simulink model "car"  (R2020a)
settings: Solver=FixedStepDiscrete  StartTime=0.0  StopTime=10.0  FixedStep=0.01  RelTol=1e-3
undefined symbols (not defined in the file or in its folder): f, Gain
libraries: instrumentlib x2
settings Model: Creator=K7050  LastModifiedBy=K7050

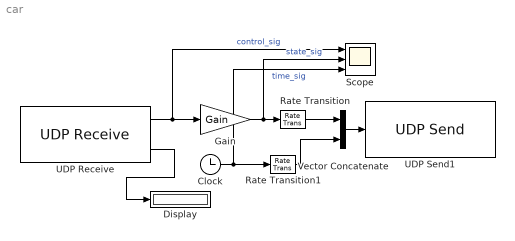
== system car ==
  Clock : Clock
  Display : Display
  Gain : Gain  Gain=Gain
  Rate Transition : RateTransition  OutPortSampleTime=0.01
  Rate Transition1 : RateTransition  OutPortSampleTime=0.01
  Scope : Scope  NumInputPorts=3
  UDP Receive : instrumentlib/UDP Receive  Host=127.0.0.1  Port=12349  LocalPort=12345  EnablePortSharing=off  GetLatestData=off  DataSize=1  DataType=double  ASCIIFormatting=%f,  Terminator=LF  ByteOrder=LittleEndian  EnableBlockingMode=off  Timeout=10  SampleTime=0.01  LocalAddress=127.0.0.1
  UDP Send1 : instrumentlib/UDP Send  Host=127.0.0.1  Port=12346  LocalPort=12351  EnablePortSharing=off  ByteOrder=LittleEndian  OutputDatagramPacketSize=16  EnableBlockingMode=off  LocalAddress=127.0.0.1
  Vector Concatenate : Concatenate
  wires:
  UDP Receive/1 -> Scope/1, Gain/1  "control_sig"
  Vector Concatenate/1 -> UDP Send1/1
  Gain/1 -> Scope/2, Rate Transition/1  "state_sig"
  Clock/1 -> Rate Transition1/1, Scope/3  "time_sig"
  Rate Transition/1 -> Vector Concatenate/1
  Rate Transition1/1 -> Vector Concatenate/2
  UDP Receive/2 -> Display/1
